simulink model "simmodel"  (Simulink 7.8)
settings: Solver=ode45  StartTime=0.0  StopTime=Inf  RelTol=1e-3
undefined symbols (not defined in the file or in its folder): f
libraries: simulink x1
settings Model: Creator=roel  LastModifiedBy=roel

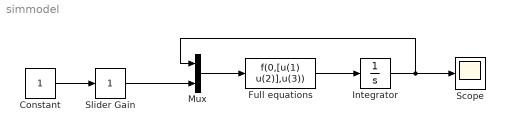
== system simmodel ==
  Constant : Constant
  Full equations : MATLABFcn  MATLABFcn=f(0,[u(1) u(2)],u(3))  OutputDimensions=2
  Integrator : Integrator  InitialCondition=[1 0]'
  Mux : Mux  Inputs=2
  Scope : Scope
      settings: YMin=-20  YMax=20
  Slider Gain : simulink/Math Operations/Slider Gain  low=0  gain=1  high=2
  wires:
  Mux/1 -> Full equations/1
  Full equations/1 -> Integrator/1
  Integrator/1 -> Scope/1, Mux/1
  Slider Gain/1 -> Mux/2
  Constant/1 -> Slider Gain/1
